simulink model "hoffmansubsystem"  (R2017a)
settings: Solver=FixedStepAuto  StartTime=0.0  StopTime=inf  RelTol=1e-3  EnableMultiTasking=on
model workspace: external: MATLAB File (data not in the file)
undefined symbols (not defined in the file): Angular, Linear, Pose
libraries: robotlib x11, aerolibtransform2 x2
settings Model: Creator=ece446  LastModifiedBy=ece446
settings OptimizationCC: DefaultUnderspecifiedDataType=single  LifeSpan=Inf  MaxStackSize=64
settings DebuggingCC: SFUnexpectedBacktrackingDiag=warning  SFNoUnconditionalDefaultTransitionDiag=warning  SFExecutionAtInitializationDiag=none
settings HardwareCC: ProdBitPerInt=16  ProdBitPerPointer=16  ProdBitPerSizeT=32  ProdBitPerPtrDiffT=32  ProdLargestAtomicFloat=None  ProdIntDivRoundTo=Undefined  ProdEndianess=Unspecified  ProdWordSize=16  ProdHWDeviceType=Generic->Unspecified (assume 32-bit Generic)  UseEmbeddedCoderFeatures=off
settings ModelReferenceCC: UpdateModelReferenceTargets=Force
settings RTWCC: SystemTargetFile=ert.tlc  HardwareBoard=Robot Operating System (ROS)  TLCOptions=-aInlineSetEventsForThisBaseRateFcn=TLC_FALSE -aSuppressMultiTaskScheduler=TLC_FALSE -aRateBasedStepFcn=0  TemplateMakefile=ert_default_tmf  Description=Embedded Coder  GenerateReport=on  Toolchain=Catkin  LaunchReport=on  TargetLang=C++
settings CodeAppCC: ForceParamTrailComments=on  OperatorAnnotations=on  MATLABSourceComments=on
settings ERTTargetCC: MultiwordLength=2048  ERTCustomFileBanners=off  SupportContinuousTime=on  SupportNonInlinedSFcns=on  RemoveResetFunc=off  SupportVariableSizeSignals=on  ModelStepFunctionPrototypeControlCompliant=off
settings ConfigComp: CovMetricSettings=dw  CovHtmlReporting=on  CovSaveCumulativeToWorkspaceVar=on  CovSaveSingleToWorkspaceVar=on  CovExternalEMLEnable=off

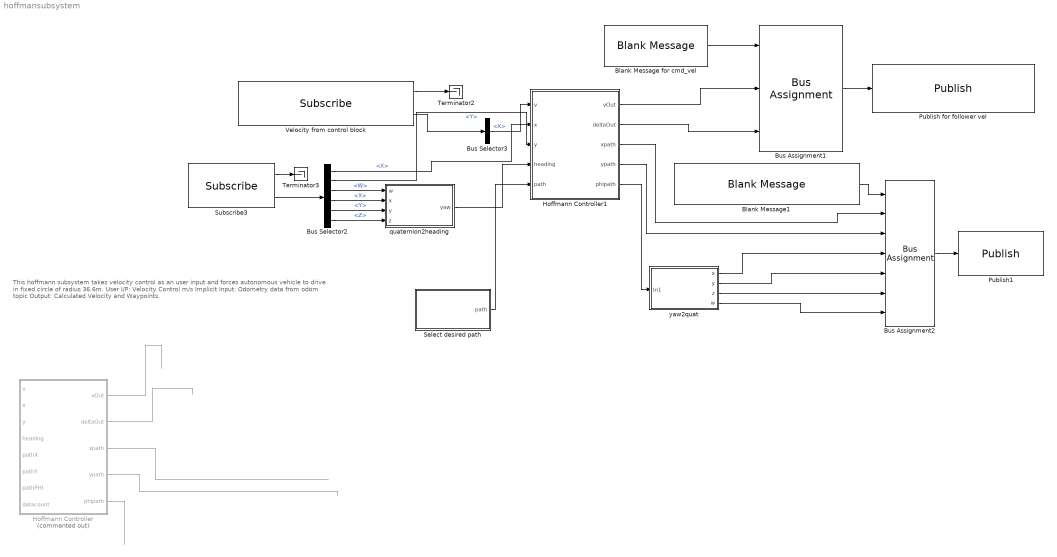
== system hoffmansubsystem ==
  note: This hoffmann subsystem takes velocity control as an user input and forces
      | autonomous vehicle to drive in fixed circle of radius 36.6m.
      | User I/P: Velocity Control m/s
      | Implicit Input: Odometry data from odom topic
      | Output: Calculated Velocity and Waypoints.
  Blank Message for cmd_vel : robotlib/Blank Message  SourceLibraryInfo=This block requires Robotics System Toolbox  messageType=geometry_msgs/Twist  SampleTime=inf
      settings: SourceProductBaseCode=RO
  Blank Message1 : robotlib/Blank Message  SourceLibraryInfo=This block requires Robotics System Toolbox  messageType=visualization_msgs/InteractiveMarkerPose  SampleTime=inf
      settings: SourceProductBaseCode=RO
  Bus Assignment1 : BusAssignment  AssignedSignals=Linear.X,Angular.Z
  Bus Assignment2 : BusAssignment  AssignedSignals=Pose.Position.X,Pose.Position.Y,Pose.Orientation.X,Pose.Orientation.Y,Pose.Orientation.Z,Pose.Orientation.W
  Bus Selector2 : BusSelector  OutputSignals=Pose.Pose.Position.X,Pose.Pose.Position.Y,Pose.Pose.Orientation.W,Pose.Pose.Orientation.X,Pose.Pose.Orientation.Y,Pose.Pose.Orientation.Z
  Bus Selector3 : BusSelector  OutputSignals=Linear.X
  Hoffmann Controller : Subsystem  Commented=on
  Hoffmann Controller1 : Subsystem
  Publish for follower vel : robotlib/Publish  SourceLibraryInfo=This block requires Robotics System Toolbox  topicSource=Specify your own  topic=cmd_vel  messageType=geometry_msgs/Twist  messageQueueLength=1
      settings: SourceProductBaseCode=RO
  Publish1 : robotlib/Publish  SourceLibraryInfo=This block requires Robotics System Toolbox  topicSource=Specify your own  topic=waypoint  messageType=visualization_msgs/InteractiveMarkerPose  messageQueueLength=1
      settings: SourceProductBaseCode=RO
  Select desired path : Subsystem
  Subscribe3 : robotlib/Subscribe  SourceLibraryInfo=This block requires Robotics System Toolbox  topicSource=Specify your own  topic=odom  messageType=nav_msgs/Odometry  sampleTime=-1  messageQueueLength=1
      settings: SourceProductBaseCode=RO
  Terminator2 : Terminator
  Terminator3 : Terminator
  "Velocity from control block " : robotlib/Subscribe  SourceLibraryInfo=This block requires Robotics System Toolbox  topicSource=Specify your own  topic=cmd_control_vel  messageType=geometry_msgs/Twist  sampleTime=-1  messageQueueLength=1
      settings: SourceProductBaseCode=RO
  quaternion2heading : Subsystem
  yaw2quat : Subsystem
  wires:
  Blank Message for cmd_vel/1 -> Bus Assignment1/1
  Bus Assignment1/1 -> Publish for follower vel/1
  Hoffmann Controller/2(deltaOut) -> ?
  Subscribe3/1 -> Terminator3/1
  Subscribe3/2 -> Bus Selector2/1
  Bus Selector2/1 -> Hoffmann Controller1/2(x)  "<X>"
  Bus Selector2/2 -> Hoffmann Controller1/3(y)  "<Y>"
  Blank Message1/1 -> Bus Assignment2/1
  Bus Assignment2/1 -> Publish1/1
  Hoffmann Controller/3(xpath) -> ?
  Hoffmann Controller/4(ypath) -> ?
  Hoffmann Controller/5(phipath) -> ?
  yaw2quat/1(x) -> Bus Assignment2/4
  yaw2quat/2(y) -> Bus Assignment2/5
  yaw2quat/3(z) -> Bus Assignment2/6
  yaw2quat/4(w) -> Bus Assignment2/7
  quaternion2heading/1(yaw) -> Hoffmann Controller1/4(heading)
  Bus Selector2/3 -> quaternion2heading/1(w)  "<W>"
  Bus Selector2/4 -> quaternion2heading/2(x)  "<X>"
  Bus Selector2/5 -> quaternion2heading/3(y)  "<Y>"
  Bus Selector2/6 -> quaternion2heading/4(z)  "<Z>"
  "Velocity from control block "/2 -> Bus Selector3/1
  "Velocity from control block "/1 -> Terminator2/1
  Bus Selector3/1 -> Hoffmann Controller1/1(v)  "<X>"
  Hoffmann Controller/1(vOut) -> ?
  Select desired path/1(path) -> Hoffmann Controller1/5(path)
  Hoffmann Controller1/1(vOut) -> Bus Assignment1/2
  Hoffmann Controller1/2(deltaOut) -> Bus Assignment1/3
  Hoffmann Controller1/3(xpath) -> Bus Assignment2/2
  Hoffmann Controller1/4(ypath) -> Bus Assignment2/3
  Hoffmann Controller1/5(phipath) -> yaw2quat/1(In1)

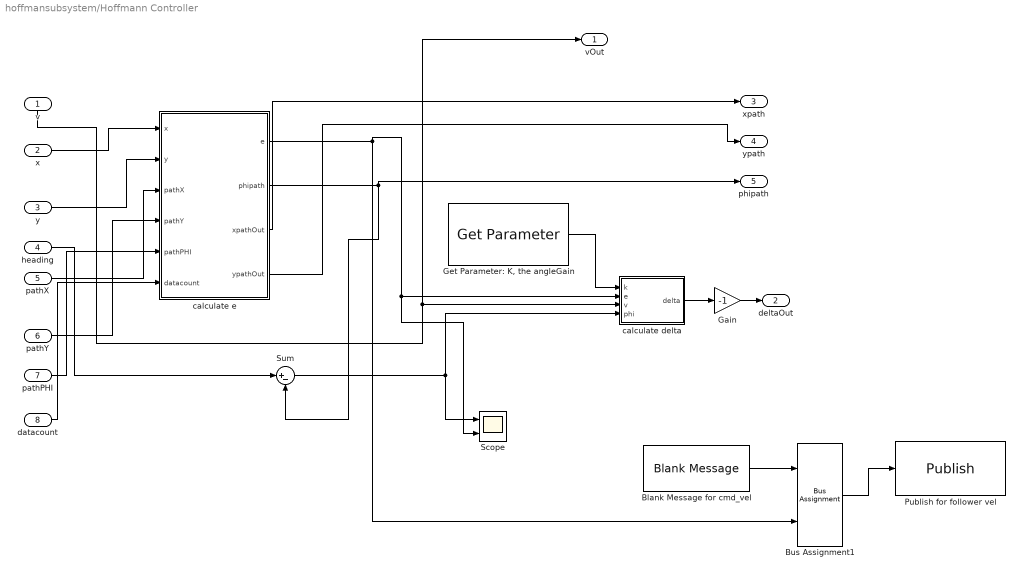
== system hoffmansubsystem/Hoffmann Controller ==
  v : Inport
  x : Inport  Port=2
  y : Inport  Port=3
  heading : Inport  Port=4
  pathX : Inport  Port=5
  pathY : Inport  Port=6
  pathPHI : Inport  Port=7
  datacount : Inport  Port=8
  Blank Message for cmd_vel : robotlib/Blank Message  SourceLibraryInfo=This block requires Robotics System Toolbox  messageType=std_msgs/Float64  SampleTime=inf
      settings: SourceProductBaseCode=RO
  Bus Assignment1 : BusAssignment  AssignedSignals=Data
  Gain : Gain  Gain=-1
  "Get Parameter: K, the angleGain" : robotlib/Get Parameter  SourceLibraryInfo=This block requires Robotics System Toolbox  ParameterSource=Specify your own  ParameterName=/azcar_sim/angleGain  ParameterType=double  ParameterMaxArrayLength=32000  ParameterInitialValue=1.0  SampleTime=-1  ShowErrorCodeOutput=off  ModelName=hoffmansubsystem  BlockId=ParamGet_hoffmansubsystem_259
      settings: SourceProductName=Robotics System Toolbox  SourceProductBaseCode=RO
  Publish for follower vel : robotlib/Publish  SourceLibraryInfo=This block requires Robotics System Toolbox  topicSource=Specify your own  topic=/azcar_sim/error  messageType=std_msgs/Float64  messageQueueLength=1
      settings: SourceProductBaseCode=RO
  Scope : Scope  NumInputPorts=2
  Sum : Sum  Inputs=|+-
  calculate delta : MATLAB Function  TreatAsAtomicUnit=on
  calculate e : MATLAB Function  TreatAsAtomicUnit=on
  vOut : Outport
  deltaOut : Outport  Port=2
  xpath : Outport  Port=3
  ypath : Outport  Port=4
  phipath : Outport  Port=5
  wires:
  v/1 -> vOut/1, calculate delta/3(v)
  pathX/1 -> calculate e/3(pathX)
  x/1 -> calculate e/1(x)
  y/1 -> calculate e/2(y)
  calculate e/2(phipath) -> Sum/2, phipath/1
  calculate e/1(e) -> Scope/2, calculate delta/2(e), Bus Assignment1/2
  Sum/1 -> Scope/1, calculate delta/4(phi)
  "Get Parameter: K, the angleGain"/1 -> calculate delta/1(k)
  calculate e/3(xpathOut) -> xpath/1
  calculate e/4(ypathOut) -> ypath/1
  heading/1 -> Sum/1
  calculate delta/1(delta) -> Gain/1
  Gain/1 -> deltaOut/1
  Blank Message for cmd_vel/1 -> Bus Assignment1/1
  Bus Assignment1/1 -> Publish for follower vel/1
  pathY/1 -> calculate e/4(pathY)
  pathPHI/1 -> calculate e/5(pathPHI)
  datacount/1 -> calculate e/6(datacount)

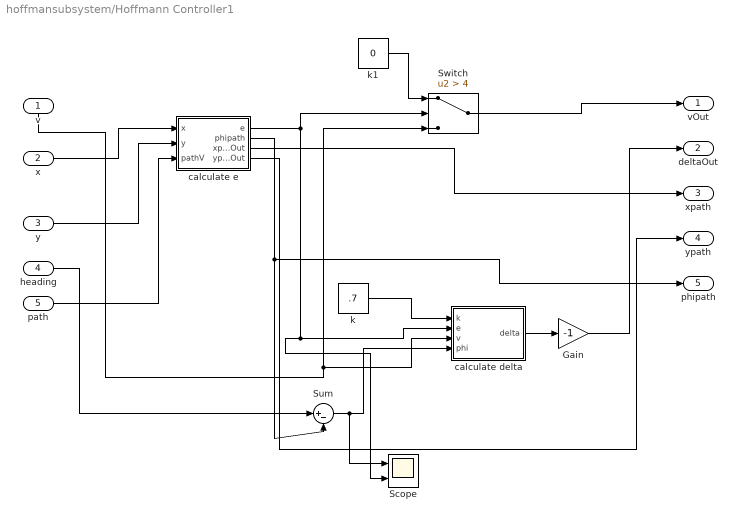
== system hoffmansubsystem/Hoffmann Controller1 ==
  v : Inport
  x : Inport  Port=2
  y : Inport  Port=3
  heading : Inport  Port=4
  path : Inport  Port=5
  Gain : Gain  Gain=-1
  Scope : Scope  NumInputPorts=2
  Sum : Sum  Inputs=|+-
  Switch : Switch  Criteria=u2 > Threshold  Threshold=4
  calculate delta : MATLAB Function  TreatAsAtomicUnit=on
  calculate e : MATLAB Function  TreatAsAtomicUnit=on
  k : Constant  Value=.7
  k1 : Constant  Value=0
  vOut : Outport
  deltaOut : Outport  Port=2
  xpath : Outport  Port=3
  ypath : Outport  Port=4
  phipath : Outport  Port=5
  wires:
  v/1 -> Switch/3, calculate delta/3(v)
  path/1 -> calculate e/3(pathV)
  x/1 -> calculate e/1(x)
  y/1 -> calculate e/2(y)
  calculate e/2(phipath) -> phipath/1, Sum/2
  calculate e/1(e) -> Switch/2, Scope/2, calculate delta/2(e)
  Sum/1 -> Scope/1, calculate delta/4(phi)
  k/1 -> calculate delta/1(k)
  calculate e/3(xpathOut) -> xpath/1
  calculate e/4(ypathOut) -> ypath/1
  Switch/1 -> vOut/1
  k1/1 -> Switch/1
  heading/1 -> Sum/1
  calculate delta/1(delta) -> Gain/1
  Gain/1 -> deltaOut/1

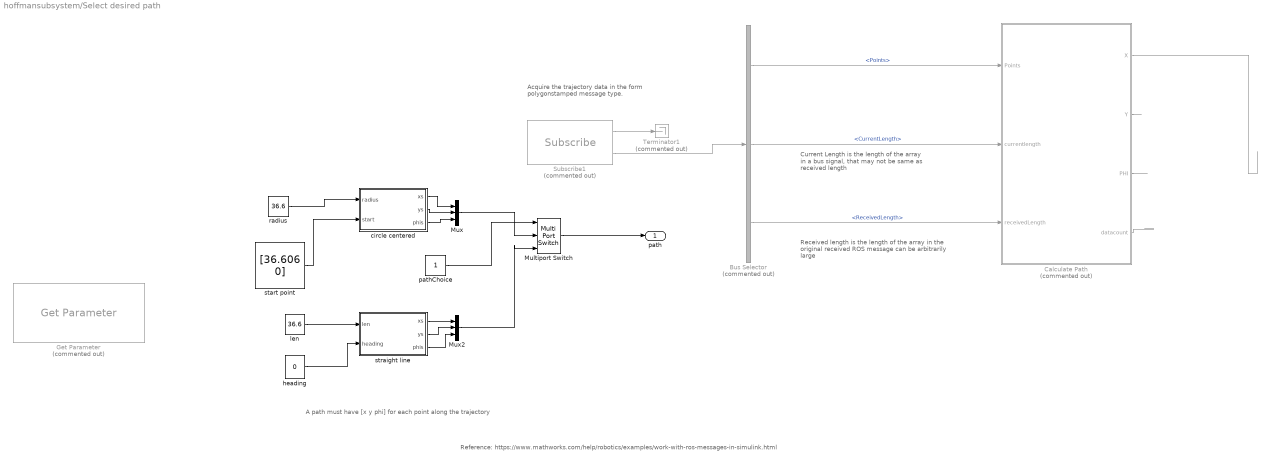
== system hoffmansubsystem/Select desired path ==
  note: Reference: https://www.mathworks.com/help/robotics/examples/work-with-ros-messages-in-simulink.html
  note: Received length is the length of the array in
      | the original received ROS message can
      | be arbitrarily large
  note: Current Length is the length of the array in a bus signal, that may not be same as received length
  note: Acquire the trajectory data in the form polygonstamped message type.
  note: A path must have [x y phi] for each point along the trajectory
  Bus Selector : BusSelector  Commented=on  OutputSignals=Polygon.Points,Polygon.Points_SL_Info.CurrentLength,Polygon.Points_SL_Info.ReceivedLength
  Calculate Path : MATLAB Function  Commented=on  TreatAsAtomicUnit=on
  Get Parameter : robotlib/Get Parameter  Commented=on  SourceLibraryInfo=This block requires Robotics System Toolbox  ParameterSource=Specify your own  ParameterName=/azcar_sim/inputFile  ParameterType=uint8[] (string)  ParameterMaxArrayLength=32000  ParameterInitialValue=0.0  SampleTime=-1  ShowErrorCodeOutput=off  ModelName=hoffmansubsystem  BlockId=ParamGet_hoffmansubsystem_240
      settings: SourceProductName=Robotics System Toolbox  SourceProductBaseCode=RO
  Multiport Switch : MultiPortSwitch  Inputs=2
  Mux : Mux  Inputs=3
  Mux2 : Mux  Inputs=3
  Subscribe1 : robotlib/Subscribe  Commented=on  SourceLibraryInfo=This block requires Robotics System Toolbox  topicSource=Select from ROS network  topic=/trajectory  messageType=geometry_msgs/PolygonStamped  sampleTime=-1  messageQueueLength=1
      settings: SourceProductBaseCode=RO
  Terminator1 : Terminator  Commented=on
  circle centered : MATLAB Function  TreatAsAtomicUnit=on
  heading : Constant  Value=0
  len : Constant  Value=36.6
  "pathChoice " : Constant
  radius : Constant  Value=36.6
  start point : Constant  Value=[36.606 0]
  straight line : MATLAB Function  TreatAsAtomicUnit=on
  path : Outport
  wires:
  Calculate Path/1(X) -> ?
  Calculate Path/2(Y) -> ?
  Calculate Path/3(PHI) -> ?
  Calculate Path/4(datacount) -> ?
  Subscribe1/1 -> Terminator1/1
  Subscribe1/2 -> Bus Selector/1
  Bus Selector/1 -> Calculate Path/1(Points)  "<Points>"
  Bus Selector/2 -> Calculate Path/2(currentlength)  "<CurrentLength>"
  Bus Selector/3 -> Calculate Path/3(receivedLength)  "<ReceivedLength>"
  straight line/2(ys) -> Mux2/2
  radius/1 -> circle centered/1(radius)
  "pathChoice "/1 -> Multiport Switch/1
  Multiport Switch/1 -> path/1
  straight line/1(xs) -> Mux2/1
  start point/1 -> circle centered/2(start)
  circle centered/3(phis) -> Mux/3
  len/1 -> straight line/1(len)
  heading/1 -> straight line/2(heading)
  circle centered/1(xs) -> Mux/1
  circle centered/2(ys) -> Mux/2
  Mux2/1 -> Multiport Switch/3
  Mux/1 -> Multiport Switch/2
  straight line/3(phis) -> Mux2/3

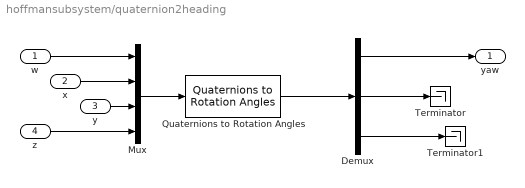
== system hoffmansubsystem/quaternion2heading ==
  w : Inport
  x : Inport  Port=2
  y : Inport  Port=3
  z : Inport  Port=4
  Demux : Demux  Outputs=3
  Mux : Mux
  Quaternions to Rotation Angles : aerolibtransform2/Quaternions to Rotation Angles  rotationOrder=ZYX
      settings: SourceProductName=Aerospace Blockset  SourceProductBaseCode=AE
  Terminator : Terminator
  Terminator1 : Terminator
  yaw : Outport
  wires:
  Quaternions to Rotation Angles/1 -> Demux/1
  Demux/2 -> Terminator/1
  Demux/3 -> Terminator1/1
  Demux/1 -> yaw/1
  w/1 -> Mux/1
  x/1 -> Mux/2
  y/1 -> Mux/3
  z/1 -> Mux/4
  Mux/1 -> Quaternions to Rotation Angles/1

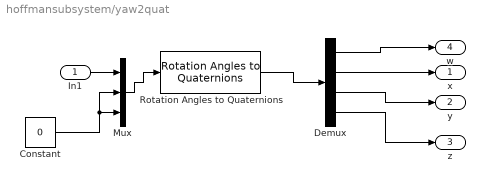
== system hoffmansubsystem/yaw2quat ==
  In1 : Inport
  Constant : Constant  Value=0
  Demux : Demux
  Mux : Mux  Inputs=3
  Rotation Angles to Quaternions : aerolibtransform2/Rotation Angles to Quaternions  rotationOrder=ZYX
      settings: SourceProductName=Aerospace Blockset  SourceProductBaseCode=AE
  x : Outport
  y : Outport  Port=2
  z : Outport  Port=3
  w : Outport  Port=4
  wires:
  Rotation Angles to Quaternions/1 -> Demux/1
  Demux/1 -> w/1
  Demux/2 -> x/1
  Demux/3 -> y/1
  Demux/4 -> z/1
  In1/1 -> Mux/1
  Mux/1 -> Rotation Angles to Quaternions/1
  Constant/1 -> Mux/3, Mux/2

== matlab function hoffmansubsystem/Hoffmann Controller/calculate e ==
  data: e output; x input; y input; pathX input; phipath output; xpathOut output; ypathOut output; pathY input; pathPHI input; datacount input
function [e,phipath,xpathOut,ypathOut] = fcn(x, y, pathX, pathY, pathPHI, datacount)
%#codegen
% path=reshape(pathV,[],3);
% x1 = pathX;
% y1 = pathY;
% phi1=pathPHI;
% 
% persistent oldPhi
% if isempty(oldPhi)
%       oldPhi = 0;
% end


etmp = inf;
e = inf;
index=1;
% find the nearest x,y on the path
for i=2:datacount
   etmp = sqrt((x-pathX(i))^2+(y-pathY(i))^2);
   if( etmp < e )
       e = etmp;
       index=i;
   end
end

xpathOut=pathX(index);
ypathOut=pathY(index);
phipath=pathPHI(index);

ex1 = (pathX(index)-x);
ey1 = (pathY(index)-y);
ex2 = cos(phipath);
ey2 = sin(phipath);
sinnnn = ex1*ey2-ey1*ex2;
e = sign(sinnnn)*e;

== matlab function hoffmansubsystem/Select desired path/Calculate Path ==
  data: X output size=32000; Points input Bus: SL_Bus_hoffmansubsystem_geometry_msgs_Point32 size=8000 [0..32000]; currentlength input; Y output size=32000; PHI output size=32000; datacount output; receivedLength input
function [X, Y,PHI,datacount] = fcn(Points, currentlength, receivedLength)
%#codegen


X = zeros(8000,1);
Y = zeros(8000,1);
PHI = zeros(8000,1);

%We will work on array using the current Length as, Simulink might
%truncate an arbitrarily large according to the maximum length set


for i = 1:currentlength
        %Points(i).X
        %Points(i).Y
        X(i) = Points(i).X;
        Y(i) = Points(i).Y;

        %We will calculate current headway as the instantaneous slope
        if ( i > 1)
           % atan2((Y(i) - Y(i-1)),(X(i) - X(i-1)))
           PHI(i) = atan2((Y(i) - Y(i-1)),(X(i) - X(i-1)));
        else
           PHI(i) = 0;
        end
end
X(i+1) =  Points(1).X;
Y(i+1) = Points(1).Y;
PHI(i+1) = atan2((Y(1) - Y(i)),(X(1) - X(i)));

datacount = double(currentlength+1);
end

== matlab function hoffmansubsystem/Hoffmann Controller/calculate delta ==
  data: delta output; k input; e input; v input; phi input
function delta = fcn(k,e,v,phi)
%#codegen
if( abs(v) < eps )
    v = eps;
end

% if phi is greater than pi (or less than -pi), then 
% we normalize to between [-pi,pi]
if( phi < -pi )
    phi = phi+2*pi;
elseif( phi > pi )
    phi = phi-2*pi;
end

% if we are pointed the "wrong" way, then screw it, let's
% follow in the direction the path is easiest to follow
% JMS I think I have a logic error here
%if( phi < -pi/2 || phi > pi/2 )
%    phi = max(min(phi - pi,pi/2),-pi/2);
%end

delta = phi + atan2(k*e,v);

== matlab function hoffmansubsystem/Select desired path/circle centered ==
  data: xs output; radius input; start input; ys output; phis output
function [xs,ys,phis] = fcn(radius,start)
%#codegen
angles=linspace(-pi,pi,301);
r = radius*exp(angles*1j);
xs = real(r)-radius+start(1);
ys = imag(r)+start(2);
phis=(pi/2)+angles;

% % To visualize the angles, run this code:
% radius=3.6; start=[0 0];
% angles=linspace(-pi,pi,300);
% r = radius*exp(angles*1j);
% xs = real(r)-radius+start(1);
% ys = imag(r)+start(2);
% % since the direction of travel is in the 'x' direction, the 
% % heading (phi) matchines the angle of the circle
% phis=(pi/2)+angles;
% xends=cos(phis);yends=sin(phis);
% figure;plot(xs,ys);hold on; quiver(xs,ys,xends,yends);axis equal;hold off

== matlab function hoffmansubsystem/Select desired path/straight line ==
  data: xs output; len input; heading input; ys output; phis output
function [xs,ys,phis] = fcn(len,heading)
%#codegen
r = linspace(0,len,301);
xs = r*cos(heading);
ys = r*sin(heading);
phis = heading*ones(1,length(r));

== matlab function hoffmansubsystem/Hoffmann Controller1/calculate delta ==
  data: delta output; k input; e input; v input; phi input
function delta = fcn(k,e,v,phi)
%#codegen
if( abs(v) < eps )
    v = eps;
end

% if phi is greater than pi (or less than -pi), then 
% we normalize to between [-pi,pi]
if( phi < -pi )
    phi = phi+2*pi;
elseif( phi > pi )
    phi = phi-2*pi;
end

delta = phi + atan2(k*e,v);

== matlab function hoffmansubsystem/Hoffmann Controller1/calculate e ==
  data: e output; x input; y input; pathV input; phipath output; xpathOut output; ypathOut output
function [e,phipath,xpathOut,ypathOut] = fcn(x,y,pathV)
%#codegen
path=reshape(pathV,[],3);
x1 = path(1,1);
y1 = path(1,2);
phi1=path(1,3);
etmp = inf;
e = inf;
index=1;
% find the nearest x,y
for i=1:length(path)
   etmp = sqrt((x-path(i,1))^2+(y-path(i,2))^2);
   if( etmp < e )
       e = etmp;
       index=i;
   end
end

xpathOut=path(index,1);
ypathOut=path(index,2);
phipath=path(index,3);

ex1 = (path(index,1)-x);
ey1 = (path(index,2)-y);
ex2 = cos(phipath);
ey2 = sin(phipath);
sinnnn = ex1*ey2-ey1*ex2;
e = sign(sinnnn)*e;
